simulink model "lib_TorqueDistribution_StateFlow_2015b-Ghost"  (R2016b)
settings: Solver=VariableStepAuto  StartTime=0.0  StopTime=10.0  RelTol=1e-3
libraries: simulink x10
(part 3 of 3)

== stateflow chart lib_TorqueDistribution_StateFlow_2015b-Ghost/Supervisory  Control  Logic1 ==
  note: 
  state VehOn
    en:
    mode = 6;
    powerMode = 1;
    HV_Req=1;
    ClutchEngage = 2000;
  note: Tranmission Shift Level Position (ShftLvrPos):
  state VehOffOrAcc
    en:
    mode=0;
    powerMode = 0;
    EnablePrplsn = 0;
    HV_Req=0;
    closeMaincReq=0;
    ClutchEngage = 2000;
  state Close_Contactors
    en:
    closeMaincReq=1;
    ClutchEngage = 2000;
  state VehShutdown
    en:
    powerMode = 1;
    EnablePrplsn = 0;
    EngOnReq = 0;
    MotTrqReq = 0;
    EngAppReq = 0;
    EnableInverter=0;
    mode=8;
    ClutchEngage = 2000;
    closeMaincReq=0;
    HV_Req=0;
  state Charging
    en:
    mode = 9;
    powerMode = 3;
    HV_Req=1;
    closeMaincReq = 1;
    EnablePrplsn = 0;
    EnableInverter = 0;
  state EnablePropulsion
    en:
    mode=7;
    EnablePrplsn = 1;
    ClutchEngage = 2000;
  note: System Power Mode (KeyPos):
  state VehReady
    en:
    powerMode = 2;
    state EnableMotor
      EnableInverter=1;
    state Eng_Charging
      en:
      EngOnReq = 1;
      mode=5;
      du:
      MotTrqReq = MotTrqCalc(ShftLvrPos,DrvIntdAxleTrq,EngTrq);
      EngTrq = EngTrqCalc(drvAPP,EngSpd,ShftLvrPos,DrvIntdAxleTrq,TransRatio);
      EngAppReq=drvAPP;
      ClutchEngage=0;
      state Trq = EngTrqCalc(EngSpeed,APP,ShftLvrPos,DrvIntdAxleTrq,TransRatio) [function]
      state MotTrq = MotTrqCalc(ShftLvrPos,DrvIntdAxleTrq,Trq) [function]
      state APP = EngTrq2EngApp(Trq,TransRatio) [function]
    state Clutch_Engage2
      en:
      MotTrqReq = 0;
      EngAppReq = 0;
      state EngStart1
        en: EngOnReq = 1;
      state EngApp = SyncCtrl(EngSpeed,MotorSpeed) [function]
      state EngageClutch
        en:
        ClutchEngage = 0;
      state EngSpdSync
        du:
        EngAppReq = SyncCtrl(EngSpd,MotSpd);
      state EngageClutch1
        en:
        ClutchEngage = 0;
      (default) -> (junction 1938)
      (junction 1938) -> VehReady.Clutch_Engage2.EngStart1 [order 2] : [ClutchEngage == 2000]
      (junction 1938) -> VehReady.Clutch_Engage2.EngageClutch [order 1] : [ClutchEngage == 0]
      VehReady.Clutch_Engage2.EngStart1 -> VehReady.Clutch_Engage2.EngSpdSync : [EngRunAtv]
      VehReady.Clutch_Engage2.EngSpdSync -> VehReady.Clutch_Engage2.EngageClutch1
    state Eng_Only_Mode
      en:
      EngOnReq = 1;
      mode=3;
      du:
      MotTrqReq = 0;
      closeMaincReq=0;
      EngTrq = EngTrqCalc(drvAPP,EngSpd,ShftLvrPos,DrvIntdAxleTrq,TransRatio);
      EngAppReq=drvAPP;
      state T = EngTrqCalc(APP,EngSpeed,Shifter,DrvIntdAxleTrq,TransRatio) [function]
      state APP = EngTrq2EngApp(T,TransRatio) [function]
    state Clutch_Engage1
      en:
      MotTrqReq = 0;
      EngAppReq = 0;
      state EngStart1
        en: EngOnReq = 1;
      state EngApp = SyncCtrl(EngSpeed,MotorSpeed) [function]
      state EngageClutch
        en:
        ClutchEngage = 0;
      state EngSpdSync
        du:
        EngAppReq = SyncCtrl(EngSpd,MotSpd);
      state EngageClutch1
        en:
        ClutchEngage = 0;
      (default) -> (junction 1687)
      (junction 1687) -> VehReady.Clutch_Engage1.EngStart1 [order 2] : [ClutchEngage == 2000]
      (junction 1687) -> VehReady.Clutch_Engage1.EngageClutch [order 1] : [ClutchEngage == 0]
      VehReady.Clutch_Engage1.EngStart1 -> VehReady.Clutch_Engage1.EngSpdSync : [EngRunAtv]
      VehReady.Clutch_Engage1.EngSpdSync -> VehReady.Clutch_Engage1.EngageClutch1
    state CD_Mode
      en:
      mode=1;
      state Drive_mode
        en:
        mode=11;
        Brkmode=0;
        EngOnReq=0;
        du:
        MotTrqReq = MotTrqCalc2(drvAPP,ShftLvrPos,DrvIntdAxleTrq,TransRatio);
        EngAppReq=0;
        ClutchEngage=2000;
        state MotTrq = MotTrqCalc2(APP,ShftLvrPos,DrvIntdAxleTrq,TransRatio) [function]
      state Brake_mode
        en:
        mode=12;
        EngAppReq=0;
        state Regen_mode
          en:
          Brkmode=1;
          du:
          MotTrqReq=MotTrqCalc1(BrkPdlPos,VehicleSpeed,...
          ShftLvrPos,MotSpd,TransRatio,IntdAxleTrq);
        state No_regen
          en:
          Brkmode=2;
          du:
          MotTrqReq=MotTrqCalc2(ShftLvrPos,TransRatio);
        state Temp_delay
        state Temp_delay1
        state T = MotTrqCalc1(BPP,VehSpd,ShftLvrPos,MotSpeed,TransRatio,IntdAxleTrq) [function]
        state T = MotTrqCalc2(ShftLvrPos,TransRatio) [function]
        (default) -> VehReady.CD_Mode.Brake_mode.No_regen
        VehReady.CD_Mode.Brake_mode.Regen_mode -> VehReady.CD_Mode.Brake_mode.Temp_delay : [RegenBrkDisable||SoC>=80||ABSAtv||Regen_fault]
        VehReady.CD_Mode.Brake_mode.Temp_delay -> VehReady.CD_Mode.Brake_mode.No_regen : after(0.25,sec)
        VehReady.CD_Mode.Brake_mode.Temp_delay1 -> VehReady.CD_Mode.Brake_mode.Regen_mode : after(0.25,sec)
        VehReady.CD_Mode.Brake_mode.No_regen -> VehReady.CD_Mode.Brake_mode.Temp_delay1 : [RegenBrkDisable == 0&&SoC<80&&ABSAtv==0&&Regen_fault==0]
      state Time_delay
      state Time_delay1
      (default) -> VehReady.CD_Mode.Drive_mode
      VehReady.CD_Mode.Drive_mode -> VehReady.CD_Mode.Time_delay : [BrkPdlPos>0&&IntdAxleTrq<0]
      VehReady.CD_Mode.Time_delay -> VehReady.CD_Mode.Brake_mode : after(0.25,sec)
      VehReady.CD_Mode.Time_delay1 -> VehReady.CD_Mode.Drive_mode : after(0.25,sec)
      VehReady.CD_Mode.Brake_mode -> VehReady.CD_Mode.Time_delay1 : [drvAPP>0&&IntdAxleTrq>=0]
    state Sport_Mode
      en:
      mode=4;
      EngOnReq = 1;
      state Brake_mode
        du:
        EngTrq =0;
        EngAppReq = 0;
        state regen_mode
          en:
          Brkmode=1;
          du:
          MotTrqReq=MotTrqCalc1(BrkPdlPos,VehicleSpeed,...
          ShftLvrPos,MotSpd,IntdAxleTrq,TransRatio);
        state No_regen
          en:
          Brkmode=2;
          du:
          MotTrqReq=0;
        state Temp_delay
        state Temp_delay1
        state T = MotTrqCalc1(BPP,VehSpd,ShftLvrPos,MotSpeed,IntdAxleTrq,TransRatio) [function]
        (default) -> VehReady.Sport_Mode.Brake_mode.No_regen
        VehReady.Sport_Mode.Brake_mode.regen_mode -> VehReady.Sport_Mode.Brake_mode.Temp_delay : [RegenBrkDisable||SoC>=80||ABSAtv||Regen_fault]
        VehReady.Sport_Mode.Brake_mode.Temp_delay -> VehReady.Sport_Mode.Brake_mode.No_regen : after(0.5,sec)
        VehReady.Sport_Mode.Brake_mode.No_regen -> VehReady.Sport_Mode.Brake_mode.Temp_delay1 : [!RegenBrkDisable&&SoC<80&&ABSAtv==0&&!Regen_fault]
        VehReady.Sport_Mode.Brake_mode.Temp_delay1 -> VehReady.Sport_Mode.Brake_mode.regen_mode : after(1,sec)
      state Drive_mode
        du:
        MotTrqReq = MotTrqCalc(drvAPP,ShftLvrPos,MotSpd,DrvIntdAxleTrq,TransRatio);
        EngTrq = EngTrqCalc(drvAPP,EngSpd,ShftLvrPos,DrvIntdAxleTrq,TransRatio);
        EngAppReq = EngTrq2EngApp(EngTrq,TransRatio);
      state Time_delay
      state Time_delay1
      state T = MotTrqCalc(APP,Shifter,MotSpeed,DrvIntdAxleTrq,TransRatio) [function]
      state T = EngTrqCalc(APP,EngSpeed,Shifter,DrvIntdAxleTrq,TransRatio) [function]
      state APP = EngTrq2EngApp(Trq,TransRatio) [function]
      (default) -> VehReady.Sport_Mode.Drive_mode
      VehReady.Sport_Mode.Drive_mode -> VehReady.Sport_Mode.Time_delay : [BrkPdlPos>0&&IntdAxleTrq<0]
      VehReady.Sport_Mode.Time_delay -> VehReady.Sport_Mode.Brake_mode
      VehReady.Sport_Mode.Time_delay1 -> VehReady.Sport_Mode.Drive_mode
      VehReady.Sport_Mode.Brake_mode -> VehReady.Sport_Mode.Time_delay1 : [drvAPP>0&&IntdAxleTrq>=0]
    state Clutch_Engage3
      en:
      MotTrqReq = 0;
      EngAppReq = 0;
      ClutchEngage = 0;
      state EngApp = SyncCtrl(EngSpeed,MotorSpeed) [function]
      state EngStart
        en: EngOnReq = 1;
      (default) -> VehReady.Clutch_Engage3.EngStart : [VehicleSpeed < 1 && TransEstGear == 15]
    state Clutch_Engage
      en:
      MotTrqReq = 0;
      EngAppReq = 0;
      state EngStart1
        en: EngOnReq = 1;
      state EngApp = SyncCtrl(EngSpeed,MotorSpeed) [function]
      state EngageClutch
        en:
        ClutchEngage = 0;
      state EngSpdSync
        du:
        EngAppReq = SyncCtrl(EngSpd,MotSpd);
      state EngStart
        en: EngOnReq = 1;
      state EngageClutch1
        en:
        ClutchEngage = 0;
      (default) -> (junction 1792)
      (junction 1792) -> VehReady.Clutch_Engage.EngStart1 [order 2] : [VehicleSpeed >= 1]
      (junction 1792) -> VehReady.Clutch_Engage.EngageClutch [order 1] : [VehicleSpeed < 1]
      VehReady.Clutch_Engage.EngStart1 -> VehReady.Clutch_Engage.EngSpdSync : [EngRunAtv]
      VehReady.Clutch_Engage.EngageClutch -> VehReady.Clutch_Engage.EngStart : [ClutchEngage == 0]
      VehReady.Clutch_Engage.EngSpdSync -> VehReady.Clutch_Engage.EngageClutch1 : [abs(EngSpd - MotSpd) < 100]
    state CS_Mode
      state Engine_Charge
        en:
        mode=2;
        state Drive_Mode
          en:
          mode=20;
          Brkmode=0;
          du:
          EngTrq = EngTrqCalc(EngSpd,drvAPP,VehicleSpeed,ShftLvrPos,DrvIntdAxleTrq,TransRatio,SoC);
          EngAppReq = EngTrq2EngApp(EngTrq,TransRatio);
          MotTrqReq = MotTrqCalc2(drvAPP,ShftLvrPos,DrvIntdAxleTrq,TransRatio,SoC,SW_CS_ON,Faked_SoC,EngTrq,MotSpd);
          state APP = EngTrq2EngApp(Trq,TransRatio) [function]
          state Trq = EngTrqCalc(EngSpeed,APP,VehSpd,ShftLvrPos,DrvIntdAxleTrq,TransRatio,SOC) [function]
          state MotTrq = MotTrqCalc2(APP,ShftLvrPos,DrvIntdAxleTrq,TransRatio,SoC,CS_On,Faked_SoC,MotSpd,Trq) [function]
        state Brake_mode1
          en:
          mode=21;
          EngAppReq=0.51;
          state regen_mode
            en:
            Brkmode=1;
            du:
            MotTrqReq=MotTrqCalc1(BrkPdlPos,VehicleSpeed,...
            ShftLvrPos,MotSpd,TransRatio,IntdAxleTrq);
          state No_regen
            en:
            Brkmode=2;
            du:
            MotTrqReq=MotTrqCalc2(ShftLvrPos,TransRatio);
          state Temp_delay
          state Temp_delay1
          state T = MotTrqCalc1(BPP,VehSpd,ShftLvrPos,MotSpeed,TransRatio,IntdAxleTrq) [function]
          state T = MotTrqCalc2(ShftLvrPos,TransRatio) [function]
          (default) -> VehReady.CS_Mode.Engine_Charge.Brake_mode1.No_regen
          VehReady.CS_Mode.Engine_Charge.Brake_mode1.regen_mode -> VehReady.CS_Mode.Engine_Charge.Brake_mode1.Temp_delay : [RegenBrkDisable||SoC>=80||ABSAtv||Regen_fault]
          VehReady.CS_Mode.Engine_Charge.Brake_mode1.Temp_delay -> VehReady.CS_Mode.Engine_Charge.Brake_mode1.No_regen : after(0.25,sec)
          VehReady.CS_Mode.Engine_Charge.Brake_mode1.Temp_delay1 -> VehReady.CS_Mode.Engine_Charge.Brake_mode1.regen_mode : after(0.25,sec)
          VehReady.CS_Mode.Engine_Charge.Brake_mode1.No_regen -> VehReady.CS_Mode.Engine_Charge.Brake_mode1.Temp_delay1 : [RegenBrkDisable == 0&&EngSpd>1000&&SoC<80&&ABSAtv==0&&Regen_fault==0]
        state Time_delay3
        state Time_delay2
        (default) -> Drive_Mode
        Drive_Mode -> Time_delay3 : [BrkPdlPos>0 && IntdAxleTrq<0]
        Time_delay3 -> Brake_mode1 : after(0.25,sec)
        Time_delay2 -> Drive_Mode : after(0.25,sec)
        Brake_mode1 -> Time_delay2 : [drvAPP>0&&IntdAxleTrq>=0]
      state Motor_Assist
        en:
        mode=3;
        state Drive_mode
          en:
          mode=30;
          Brkmode=0;
          du:
          EngTrq = 0;
          EngAppReq = 0;
          MotTrqReq = MotTrqCalc2(drvAPP,DrvIntdAxleTrq,TransRatio,ShftLvrPos);
          state MotTrq = MotTrqCalc2(APP,DrvIntdAxleTrq,TransRatio,ShftLvrPos) [function]
        state Brake_mode
          en:
          mode=31;
          EngAppReq=0.51;
          state Regen_mode
            en:
            Brkmode=1;
            du:
            MotTrqReq=MotTrqCalc1(BrkPdlPos,VehicleSpeed,...
            ShftLvrPos,MotSpd,TransRatio,IntdAxleTrq);
          state No_regen
            en:
            Brkmode=2;
            du:
            MotTrqReq=MotTrqCalc2(ShftLvrPos,TransRatio);
          state Temp_delay
          state Temp_delay1
          state T = MotTrqCalc1(BPP,VehSpd,ShftLvrPos,MotSpeed,TransRatio,IntdAxleTrq) [function]
          state T = MotTrqCalc2(ShftLvrPos,TransRatio) [function]
          (default) -> VehReady.CS_Mode.Motor_Assist.Brake_mode.No_regen
          VehReady.CS_Mode.Motor_Assist.Brake_mode.Regen_mode -> VehReady.CS_Mode.Motor_Assist.Brake_mode.Temp_delay : [RegenBrkDisable||SoC>=80||ABSAtv||Regen_fault]
          VehReady.CS_Mode.Motor_Assist.Brake_mode.Temp_delay -> VehReady.CS_Mode.Motor_Assist.Brake_mode.No_regen : after(0.25,sec)
          VehReady.CS_Mode.Motor_Assist.Brake_mode.Temp_delay1 -> VehReady.CS_Mode.Motor_Assist.Brake_mode.Regen_mode : after(0.25,sec)
          VehReady.CS_Mode.Motor_Assist.Brake_mode.No_regen -> VehReady.CS_Mode.Motor_Assist.Brake_mode.Temp_delay1 : [RegenBrkDisable == 0&&EngSpd>1000&&SoC<80&&ABSAtv==0&&Regen_fault==0]
        state Time_delay
        state Time_delay1
        (default) -> VehReady.CS_Mode.Motor_Assist.Drive_mode
        VehReady.CS_Mode.Motor_Assist.Drive_mode -> VehReady.CS_Mode.Motor_Assist.Time_delay : [BrkPdlPos>0&&IntdAxleTrq<0]
        VehReady.CS_Mode.Motor_Assist.Time_delay -> VehReady.CS_Mode.Motor_Assist.Brake_mode : after(0.25,sec)
        VehReady.CS_Mode.Motor_Assist.Time_delay1 -> VehReady.CS_Mode.Motor_Assist.Drive_mode : after(0.25,sec)
        VehReady.CS_Mode.Motor_Assist.Brake_mode -> VehReady.CS_Mode.Motor_Assist.Time_delay1 : [drvAPP>0&&IntdAxleTrq>=0]
      state Time_Delay
      state Time_Delay1
      state Clutch_Engage
        en:
        MotTrqReq = 0;
        EngAppReq = 0;
        state EngApp = SyncCtrl(EngSpeed,MotorSpeed) [function]
        state EngStart1
          en: EngOnReq = 1;
        state EngSpdSync
          du:
          EngAppReq = SyncCtrl(EngSpd,MotSpd);
        state EngageClutch1
          en:
          ClutchEngage = 0;
        (default) -> VehReady.CS_Mode.Clutch_Engage.EngStart1
        VehReady.CS_Mode.Clutch_Engage.EngStart1 -> VehReady.CS_Mode.Clutch_Engage.EngSpdSync : [EngRunAtv]
        VehReady.CS_Mode.Clutch_Engage.EngSpdSync -> VehReady.CS_Mode.Clutch_Engage.EngageClutch1 : [abs(EngSpd - MotSpd) < 100]
      state Motor_Assist1 [commented out]
        en:
        mode=3;
        state Drive_mode [commented out]
          en:
          mode=30;
          Brkmode=0;
          du:
          EngTrq = EngTrqCalc(EngSpd,drvAPP,VehicleSpeed,ShftLvrPos,DrvIntdAxleTrq,TransRatio);
          EngAppReq = EngTrq2EngApp(EngTrq,TransRatio);
          MotTrqReq = MotTrqCalc2(drvAPP,EngFdbkTrq,ShftLvrPos,DrvIntdAxleTrq,TransRatio,EngTrq);
          state APP = EngTrq2EngApp(Trq,TransRatio) [function] [commented out]
          state MotTrq = MotTrqCalc2(APP,EngFdbkTrq,ShftLvrPos,DrvIntdAxleTrq,TransRatio,Trq) [function] [commented out]
          state Trq = EngTrqCalc(EngSpeed,APP,VehSpd,ShftLvrPos,DrvIntdAxleTrq,TransRatio) [function] [commented out]
        state Brake_mode [commented out]
          en:
          mode=31;
          EngAppReq=0.51;
          state Regen_mode [commented out]
            en:
            Brkmode=1;
            du:
            MotTrqReq=MotTrqCalc1(BrkPdlPos,VehicleSpeed,...
            ShftLvrPos,MotSpd,TransRatio,IntdAxleTrq);
          state No_regen [commented out]
            en:
            Brkmode=2;
            du:
            MotTrqReq=MotTrqCalc2(ShftLvrPos,TransRatio);
          state Temp_delay [commented out]
          state Temp_delay1 [commented out]
          state T = MotTrqCalc1(BPP,VehSpd,ShftLvrPos,MotSpeed,TransRatio,IntdAxleTrq) [function] [commented out]
          state T = MotTrqCalc2(ShftLvrPos,TransRatio) [function] [commented out]
          (default) -> VehReady.CS_Mode.Motor_Assist1.Brake_mode.No_regen [commented out]
          VehReady.CS_Mode.Motor_Assist1.Brake_mode.Regen_mode -> VehReady.CS_Mode.Motor_Assist1.Brake_mode.Temp_delay [commented out] : [RegenBrkDisable||SoC>=80||ABSAtv||Regen_fault]
          VehReady.CS_Mode.Motor_Assist1.Brake_mode.Temp_delay -> VehReady.CS_Mode.Motor_Assist1.Brake_mode.No_regen [commented out] : after(0.25,sec)
          VehReady.CS_Mode.Motor_Assist1.Brake_mode.Temp_delay1 -> VehReady.CS_Mode.Motor_Assist1.Brake_mode.Regen_mode [commented out] : after(0.25,sec)
          VehReady.CS_Mode.Motor_Assist1.Brake_mode.No_regen -> VehReady.CS_Mode.Motor_Assist1.Brake_mode.Temp_delay1 [commented out] : [RegenBrkDisable == 0&&EngSpd>1000&&SoC<80&&ABSAtv==0&&Regen_fault==0]
        state Time_delay [commented out]
        state Time_delay1 [commented out]
        (default) -> VehReady.CS_Mode.Motor_Assist1.Drive_mode [commented out]
        VehReady.CS_Mode.Motor_Assist1.Drive_mode -> VehReady.CS_Mode.Motor_Assist1.Time_delay [commented out] : [BrkPdlPos>0&&IntdAxleTrq<0]
        VehReady.CS_Mode.Motor_Assist1.Time_delay -> VehReady.CS_Mode.Motor_Assist1.Brake_mode [commented out] : after(0.25,sec)
        VehReady.CS_Mode.Motor_Assist1.Time_delay1 -> VehReady.CS_Mode.Motor_Assist1.Drive_mode [commented out] : after(0.25,sec)
        VehReady.CS_Mode.Motor_Assist1.Brake_mode -> VehReady.CS_Mode.Motor_Assist1.Time_delay1 [commented out] : [drvAPP>0&&IntdAxleTrq>=0]
      (default) -> Engine_Charge
      Engine_Charge -> Time_Delay : [(SW_CS_ON==0&&SoC > CS_SOC_MAX) || (SW_CS_ON==0&&VehicleSpeed >40 &&...
          |  SoC > (CS_SOC_MIN+5))||(SW_CS_ON&&SoC>(Faked_SoC+5))]
      Time_Delay -> Motor_Assist : after(1,sec)
      Time_Delay1 -> Engine_Charge : after(1,sec)
      Motor_Assist -> VehReady.CS_Mode.Clutch_Engage : [SoC < CS_SOC_MIN&& BrkPdlPos == 0||...
          | (SW_CS_ON&&SoC<Faked_SoC)]
      VehReady.CS_Mode.Clutch_Engage -> Time_Delay1 : [ClutchEngage==1]
    (default) -> EnableMotor : [eSystemStatus>1||...
        | iceSystemStatus>1]
    EnableMotor -> (junction 1935)
    Clutch_Engage2 -> Eng_Charging : after(1,sec)
        | [ClutchEngage==0&&...
        | EngRunAtv == 1]
    (junction 1935) -> Clutch_Engage2 [order 2] : [SW_Engine_ON&&...
        | HoodStatus==0]
    (junction 1935) -> CD_Mode [order 1] : [InverterEnabled==8&&!SW_Engine_ON]
        | {ClutchEngage = 2000;}
    CD_Mode -> Clutch_Engage1 [order 2] : [(SoC < 0.05 && ...
        | iceSystemStatus == 2)||...
        | (iceSystemStatus==2&&eSystemStatus == 0)]
    Clutch_Engage1 -> Eng_Only_Mode : after(1,sec)
        | [ClutchEngage==0&&...
        | EngRunAtv == 1]
    CD_Mode -> Clutch_Engage3 [order 3] : [SportModeEnabled == 1&&...
        | iceSystemStatus>1&&eSystemStatus>1]
    Clutch_Engage3 -> Sport_Mode : [EngRunAtv]
    Eng_Only_Mode -> CD_Mode [order 2] : [(SoC > CD_SOC_MIN && ...
        | eSystemStatus == 2) || ...
        | (iceSystemStatus == 0&&eSystemStatus)]
    Sport_Mode -> CD_Mode [order 1] : [SportModeEnabled == 0&&iceSystemStatus&&eSystemStatus]
    Eng_Only_Mode -> CS_Mode [order 1] : [SoC<CS_SOC_MIN&&SoC>0.1]
    CS_Mode -> Eng_Only_Mode [order 2] : [SoC < 0.1]
    CS_Mode -> Sport_Mode [order 1] : [SportModeEnabled == 1&&...
        | iceSystemStatus&&eSystemStatus]
    Sport_Mode -> CS_Mode [order 2] : [SportModeEnabled == 0&&...
        | iceSystemStatus&&eSystemStatus]
    CD_Mode -> VehReady.Clutch_Engage [order 1] : [(SW_CS_ON&&iceSystemStatus && ...
        | eSystemStatus)||...
        | SoC <CS_SOC_MIN&&iceSystemStatus == 2 && ...
        | eSystemStatus == 2]
    CS_Mode -> CD_Mode [order 3] : [(!SW_CS_ON&&SoC > CD_SOC_MIN&&...
        | eSystemStatus == 2) || ...
        | iceSystemStatus == 0]
    VehReady.Clutch_Engage -> CS_Mode : after(1,sec)
        | [ClutchEngage==0&&...
        | EngRunAtv == 1]
  VehOffOrAcc -> EnablePropulsion [order 3] : [KeyPos==3&&BrkPdlPos>10&&ShftLvrPos==1&&(~eSystemStatus&&iceSystemStatus)]
  (default) -> VehOffOrAcc
  VehOffOrAcc -> VehOn [order 2] : [KeyPos>= 1&&(eSystemStatus||iceSystemStatus)]
  Close_Contactors -> VehOffOrAcc [order 3] : [KeyPos < 1]
  VehOffOrAcc -> Charging [order 1] : [plugged]
  Charging -> VehOffOrAcc [order 2] : [plugged==0&&...
      | KeyPos==0]
  VehOn -> Close_Contactors : [INV_State==3]
  VehShutdown -> VehOffOrAcc [order 2] : after(1,sec)[plugged==0]
  Charging -> Close_Contactors [order 1] : [plugged==0&&...
      | KeyPos==1]
  Close_Contactors -> Charging [order 2] : [plugged]
  Close_Contactors -> EnablePropulsion [order 1] : [KeyPos==3&&BrkPdlPos>10&&...
      | ShftLvrPos==1]
  EnablePropulsion -> Charging [order 2] : [plugged]
  VehShutdown -> Charging [order 1] : [plugged]
  EnablePropulsion -> VehReady [order 1] : after(0.5,sec)
  VehReady -> Charging [order 1] : [plugged]
  VehReady -> VehShutdown [order 2] : [KeyPos < 2&&ShftLvrPos==1||...
      | (eSystemStatus==0&&iceSystemStatus==0)]
  data: Trq function_output; EngSpeed function_input; APP function_input; ShftLvrPos function_input; DrvIntdAxleTrq function_input; TransRatio function_input; MotTrq function_output; ShftLvrPos function_input; DrvIntdAxleTrq function_input; Trq function_input; Trq function_input; APP function_output; TransRatio function_input; EngSpeed function_input; EngApp function_output; MotorSpeed function_input; APP function_input; EngSpeed function_input; T function_output; Shifter function_input; DrvIntdAxleTrq function_input; TransRatio function_input; T function_input; APP function_output; TransRatio function_input; EngSpeed function_input; EngApp function_output; MotorSpeed function_input; APP function_input; MotTrq function_output; ShftLvrPos function_input; DrvIntdAxleTrq function_input; TransRatio function_input; T function_output; BPP function_input; VehSpd function_input; ShftLvrPos function_input; MotSpeed function_input; TransRatio function_input; IntdAxleTrq function_input; T function_output; ShftLvrPos function_input; TransRatio function_input; T function_output; BPP function_input; VehSpd function_input; ShftLvrPos function_input; MotSpeed function_input; IntdAxleTrq function_input; TransRatio function_input; T function_output; APP function_input; Shifter function_input; MotSpeed function_input; DrvIntdAxleTrq function_input; TransRatio function_input; APP function_input; EngSpeed function_input; T function_output; Shifter function_input; DrvIntdAxleTrq function_input; TransRatio function_input; Trq function_input; APP function_output; TransRatio function_input; temp local double; EngSpeed function_input; EngApp function_output; MotorSpeed function_input; EngSpeed function_input; EngApp function_output; MotorSpeed function_input; Trq function_input; APP function_output; TransRatio function_input; Trq function_output; EngSpeed function_input; APP function_input; VehSpd function_input; ShftLvrPos function_input; DrvIntdAxleTrq function_input; TransRatio function_input; SOC function_input; APP function_input; MotTrq function_output; ShftLvrPos function_input; DrvIntdAxleTrq function_input; TransRatio function_input; SoC function_input; CS_On function_input; Faked_SoC function_input; MotSpd function_input; Trq function_input; T function_output; BPP function_input; VehSpd function_input; ShftLvrPos function_input; MotSpeed function_input; TransRatio function_input; IntdAxleTrq function_input; T function_output; ShftLvrPos function_input; TransRatio function_input; MotTrq function_output; APP function_input; DrvIntdAxleTrq function_input; TransRatio function_input; ShftLvrPos function_input; T function_output; BPP function_input; VehSpd function_input; ShftLvrPos function_input; MotSpeed function_input; TransRatio function_input; IntdAxleTrq function_input; T function_output; ShftLvrPos function_input; TransRatio function_input; EngSpeed function_input; EngApp function_output; MotorSpeed function_input; Trq function_input double size=1; APP function_output double size=1; TransRatio function_input double size=1; APP function_input double size=1; EngFdbkTrq function_input double size=1; MotTrq function_output double size=1; ShftLvrPos function_input double size=1; DrvIntdAxleTrq function_input double size=1; TransRatio function_input double size=1; Trq function_input double size=1; Trq function_output double size=1; EngSpeed function_input double size=1; APP function_input double size=1; VehSpd function_input double size=1; ShftLvrPos function_input double size=1; DrvIntdAxleTrq function_input double size=1; TransRatio function_input double size=1; T function_output double size=1; BPP function_input double size=1; VehSpd function_input double size=1; ShftLvrPos function_input double size=1; MotSpeed function_input double size=1; TransRatio function_input double size=1; IntdAxleTrq function_input double size=1; T function_output double size=1; ShftLvrPos function_input double size=1; TransRatio function_input double size=1; data local double; SportModeEnabled input boolean; TransEstGear input int8; mode output int8; powerMode output int8; closeMaincReq output double; EnablePrplsn output boolean; KeyPos input int8; BrkPdlPos input double; drvAPP input double; VehicleSpeed input double; EngSpd input double; MotSpd input double; ShftLvrPos input int8; EngAppReq output double; EngOnReq output boolean; MotTrqReq output double; EnableInverter output boolean; InverterEnabled input double; plugged input double; CD_SOC_MIN input double; CS_SOC_MIN input double; CS_SOC_MAX input double; EngRunAtv input boolean; SoC input double; EngTrq output double; DrvIntdAxleTrq input double; IntdAxleTrq input double; Faked_SoC input double; TransRatio input double; HV_Req output double; SW_CS_ON input boolean; SW_Engine_ON input boolean; RegenBrkDisable input boolean; Chg output double; Brkmode output double; Drvmode output double; eSystemStatus input; iceSystemStatus input; Drv_Mode local double; ABSAtv input boolean; Regen_fault input boolean; EngFdbkTrq input double; EngCtlTmp input; ClutchEngage output double; INV_State input; HoodStatus input
